simulink model "Two_tank_series_Example2_1_realization"  (Simulink 7.6)
settings: Solver=ode45  StartTime=0.0  StopTime=20  RelTol=1e-3
Description:
  | Lecture 2. State space realization with matrix representation and simple elements of gains, integrators and sumation
  | 
  | Example 2.1: Two tanks in series model with the following properties:
  | 
  | x(t)= -state of the system, level tank heights, h(t)=[h_1(t) ; h_2(t)]
  | y(t)= -system's outputs, two flows F(t)=[F_2(t);F_3(t)]
  | u(t)= - input to the system, flow F_1(t)
  | 
  | The matrices describing the state space are given as follows:
  | 
  | A=[-1/A_1k_1 0;1/A_2k_1 -1/A_2k_2];
  | B=[1/A_1;0];
  | C=[1/k_1 0; 0 1/k_2];
  | D=[0;0]
  | 
  | A_1=10;  A_2=7;
  | k_1=1;    k_2=3;
  | 
  | WE CONSTRUCT THE STATE SPACE REALIZATION WITH SIMPLE ELEMENTS OF GAINS,
  | SUMATIONS AND INTEGRATORS.
  | 
  | It can be demonstrated that under the same input two realizations are identical.
settings Model: Creator=administrator  LastModifiedBy=administrator

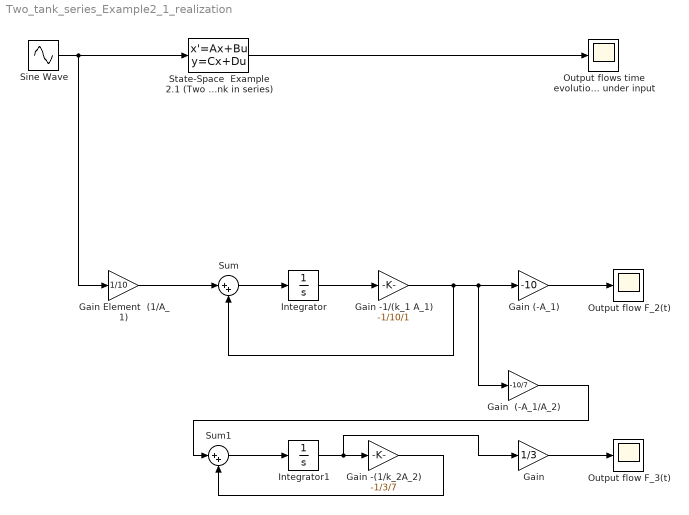
== system Two_tank_series_Example2_1_realization ==
  Gain : Gain  Gain=1/3
  Gain  (-A_1/A_2) : Gain  Gain=-10/7
  Gain (-A_1) : Gain  Gain=-10
  Gain -(1/k_2A_2) : Gain  Gain=-1/3/7
  Gain -1/(k_1 A_1) : Gain  Gain=-1/10/1
  Gain Element  (1/A_1) : Gain  Gain=1/10
  Integrator : Integrator
  Integrator1 : Integrator
  Output flow F_2(t) : Scope
      settings: TimeRange=20  YMin=-0.2  YMax=0.5
  Output flow F_3(t) : Scope
      settings: TimeRange=20  YMin=0  YMax=0.06  SaveName=ScopeData2
  Output flows time evolution under input : Scope
      settings: TimeRange=20  YMin=-0.2  YMax=0.5
  Sine Wave : Sin  Amplitude=2  SampleTime=0
  State-Space  Example 2.1 (Two tank in series) : StateSpace  A="[-1/10/1 0;1/7/1  -1/7/3]"  B=[1/10 ;0]  C=[1/1 0; 0 1/3]  D=[0; 0]  ContinuousStateAttributes='h'
  Sum : Sum  Inputs=|++
  Sum1 : Sum  Inputs=|++
  wires:
  Sine Wave/1 -> State-Space  Example 2.1 (Two tank in series)/1, Gain Element  (1/A_1)/1
  State-Space  Example 2.1 (Two tank in series)/1 -> Output flows time evolution under input/1
  Gain Element  (1/A_1)/1 -> Sum/1
  Sum/1 -> Integrator/1
  Integrator/1 -> Gain -1/(k_1 A_1)/1
  Gain -1/(k_1 A_1)/1 -> Sum/2, Gain (-A_1)/1, Gain  (-A_1/A_2)/1
  Gain (-A_1)/1 -> Output flow F_2(t)/1
  Gain  (-A_1/A_2)/1 -> Sum1/1
  Sum1/1 -> Integrator1/1
  Integrator1/1 -> Gain -(1/k_2A_2)/1, Gain/1
  Gain -(1/k_2A_2)/1 -> Sum1/2
  Gain/1 -> Output flow F_3(t)/1
